simulink model "SPK_TMT_MophongSMC_4DOF"  (R2017b)
settings: Solver=FixedStepAuto  StartTime=0.0  StopTime=100  FixedStep=0.01  RelTol=1e-3
settings Model: Creator=DELL  LastModifiedBy=DELL

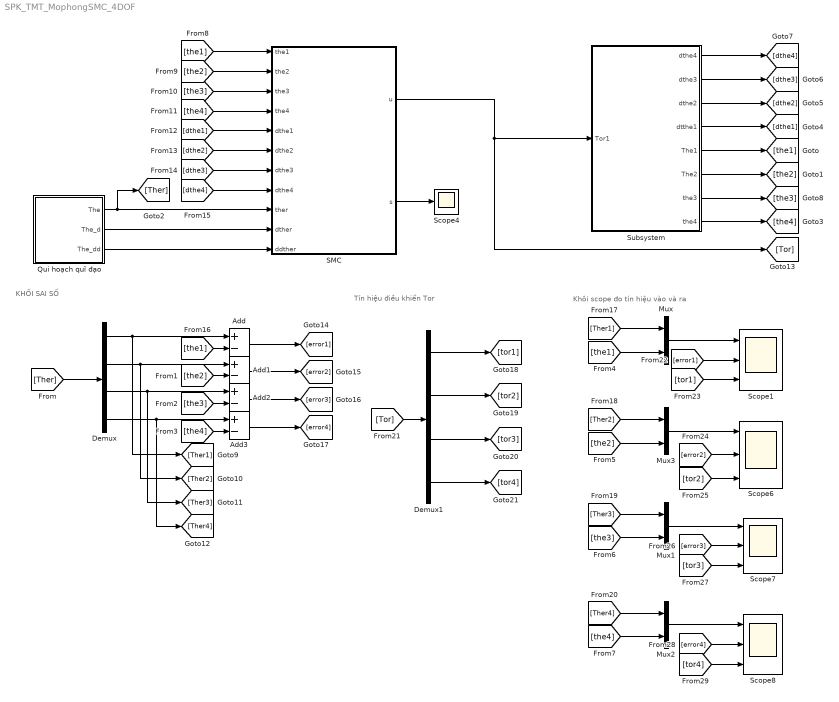
== system SPK_TMT_MophongSMC_4DOF ==
  note: Tín hiệu điều khiển Tor
  note: Khôi scope đo tín hiệu vào và ra
  note: KHỐI SAI SỐ
  Add{,1..3} (4 alike) : Sum  Inputs=+-
  Demux : Demux
  Demux1 : Demux
  Mux{,1..3} (4 alike) : Mux  Inputs=2
  "Qui hoạch quĩ đạo " : Subsystem
  SMC : MATLAB Function  TreatAsAtomicUnit=on
  Scope{1,6..8} (4 alike) : Scope  NumInputPorts=3
  Scope4 : Scope
  Subsystem : Subsystem
  wires:
  "Qui hoạch quĩ đạo "/1(The) -> [Ther], SMC/9(ther)
  "Qui hoạch quĩ đạo "/2(The_d) -> SMC/10(dther)
  "Qui hoạch quĩ đạo "/3(The_dd) -> SMC/11(ddther)
  [dthe1] -> SMC/5(dthe1)
  [the4] -> SMC/4(the4)
  [the2] -> SMC/2(the2)
  [dthe3] -> SMC/7(dthe3)
  [the1] -> SMC/1(the1)
  [dthe4] -> SMC/8(dthe4)
  [dthe2] -> SMC/6(dthe2)
  [the3] -> SMC/3(the3)
  SMC/2(s) -> Scope4/1
  Demux/1 -> [Ther1], Add/1
  [the1] -> Add/2
  Add/1 -> [error1]
  SMC/1(u) -> [Tor], Subsystem/1(Tor1)
  Subsystem/1(dthe4) -> [dthe4]
  Subsystem/2(dthe3) -> [dthe3]
  Subsystem/3(dthe2) -> [dthe2]
  Subsystem/4(dtthe1) -> [dthe1]
  Subsystem/8(the4) -> [the4]
  Subsystem/6(The2) -> [the2]
  Subsystem/5(The1) -> [the1]
  Subsystem/7(the3) -> [the3]
  [Ther] -> Demux/1
  Demux/2 -> [Ther2], Add1/1
  [the2] -> Add1/2
  Demux/3 -> [Ther3], Add2/1
  [the3] -> Add2/2
  Demux/4 -> [Ther4], Add3/1
  [the4] -> Add3/2
  Add1/1 -> [error2]
  Add2/1 -> [error3]
  Add3/1 -> [error4]
  [the1] -> Mux/2
  [the4] -> Mux2/2
  [Ther1] -> Mux/1
  [the2] -> Mux3/2
  [Ther2] -> Mux3/1
  [the3] -> Mux1/2
  [Ther3] -> Mux1/1
  [Ther4] -> Mux2/1
  Demux1/1 -> [tor1]
  Demux1/2 -> [tor2]
  Demux1/3 -> [tor3]
  Demux1/4 -> [tor4]
  [Tor] -> Demux1/1
  Mux/1 -> Scope1/1
  Mux3/1 -> Scope6/1
  Mux1/1 -> Scope7/1
  Mux2/1 -> Scope8/1
  [error1] -> Scope1/2
  [tor1] -> Scope1/3
  [error2] -> Scope6/2
  [tor2] -> Scope6/3
  [error3] -> Scope7/2
  [tor3] -> Scope7/3
  [error4] -> Scope8/2
  [tor4] -> Scope8/3

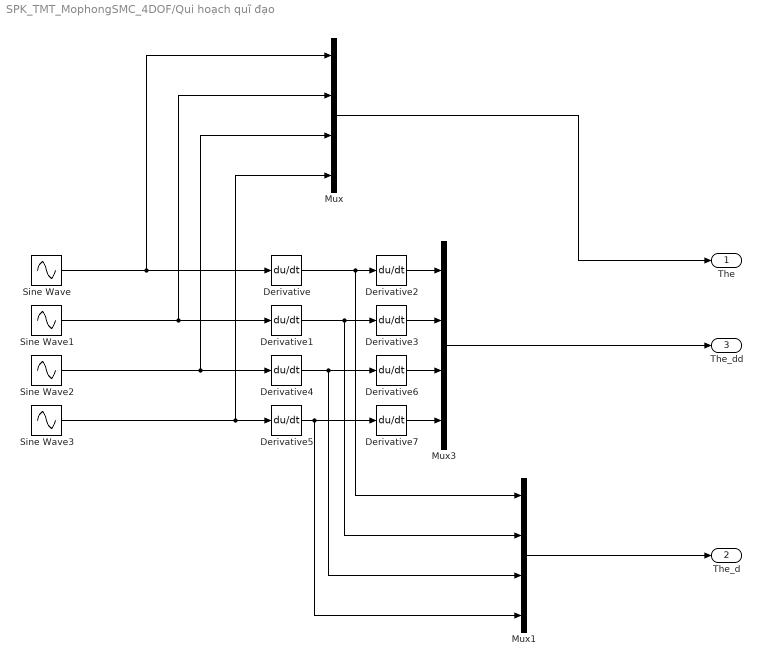
== system SPK_TMT_MophongSMC_4DOF/Qui hoạch quĩ đạo  ==
  Derivative{,1..7} (8 alike) : Derivative
  Mux : Mux
  Mux1 : Mux
  Mux3 : Mux
  Sine Wave : Sin  Amplitude=pi/6  Frequency=2*pi*0.1  SampleTime=0
  Sine Wave1 : Sin  Amplitude=pi/6  Frequency=2*pi*0.1  Phase=pi/6  SampleTime=0
  Sine Wave2 : Sin  Amplitude=pi/6  Frequency=2*pi*0.1  Phase=pi/3  SampleTime=0
  Sine Wave3 : Sin  Amplitude=pi/6  Frequency=2*pi*0.1  Phase=pi/2  SampleTime=0
  The : Outport
  The_d : Outport  Port=2
  The_dd : Outport  Port=3
  wires:
  Derivative6/1 -> Mux3/3
  Derivative7/1 -> Mux3/4
  Derivative5/1 -> Mux1/4, Derivative7/1
  Derivative4/1 -> Mux1/3, Derivative6/1
  Sine Wave2/1 -> Mux/3, Derivative4/1
  Sine Wave3/1 -> Mux/4, Derivative5/1
  Sine Wave/1 -> Mux/1, Derivative/1
  Mux1/1 -> The_d/1
  Derivative3/1 -> Mux3/2
  Derivative1/1 -> Mux1/2, Derivative3/1
  Derivative2/1 -> Mux3/1
  Sine Wave1/1 -> Mux/2, Derivative1/1
  Mux/1 -> The/1
  Mux3/1 -> The_dd/1
  Derivative/1 -> Mux1/1, Derivative2/1

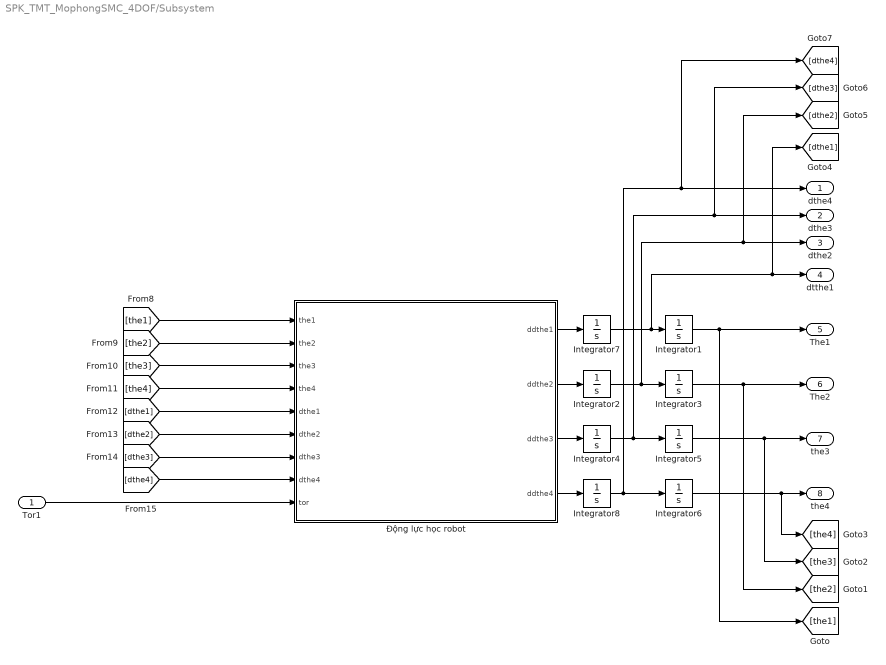
== system SPK_TMT_MophongSMC_4DOF/Subsystem ==
  Tor1 : Inport
  Integrator{1..8} (8 alike) : Integrator
  Động lực học robot : MATLAB Function  TreatAsAtomicUnit=on
  dthe4 : Outport
  dthe3 : Outport  Port=2
  dthe2 : Outport  Port=3
  dtthe1 : Outport  Port=4
  The1 : Outport  Port=5
  The2 : Outport  Port=6
  the3 : Outport  Port=7
  the4 : Outport  Port=8
  wires:
  Integrator3/1 -> [the2], The2/1
  Tor1/1 -> Động lực học robot/9(tor)
  Integrator5/1 -> [the3], the3/1
  Integrator1/1 -> [the1], The1/1
  Integrator4/1 -> [dthe3], dthe3/1, Integrator5/1
  Động lực học robot/2(ddthe2) -> Integrator2/1
  Động lực học robot/3(ddthe3) -> Integrator4/1
  Động lực học robot/4(ddthe4) -> Integrator8/1
  Integrator8/1 -> [dthe4], dthe4/1, Integrator6/1
  Động lực học robot/1(ddthe1) -> Integrator7/1
  Integrator7/1 -> [dthe1], dtthe1/1, Integrator1/1
  Integrator6/1 -> [the4], the4/1
  Integrator2/1 -> [dthe2], dthe2/1, Integrator3/1
  [dthe2] -> Động lực học robot/6(dthe2)
  [dthe4] -> Động lực học robot/8(dthe4)
  [the1] -> Động lực học robot/1(the1)
  [the2] -> Động lực học robot/2(the2)
  [the4] -> Động lực học robot/4(the4)
  [the3] -> Động lực học robot/3(the3)
  [dthe1] -> Động lực học robot/5(dthe1)
  [dthe3] -> Động lực học robot/7(dthe3)

== matlab function SPK_TMT_MophongSMC_4DOF/SMC ==
  data: the1 input; u output; the2 input; the3 input; the4 input; dthe1 input; dthe2 input; dthe3 input; dthe4 input; ther input; dther input; ddther input; s output
function [u,s]= SMC(the1, the2,the3, the4, dthe1, dthe2, dthe3, dthe4,ther,dther,ddther)
%%
m1=1;
m2=1;
m3=1;
m4=1;
L1=150;
L2=350;
L3=363.5;
L4=210;
d=140;
g=9.81;
%% M
M11=L1^2*m1 + L1^2*m2 + L1^2*m3 + (L2^2*m2)/2 + L1^2*m4 + (L2^2*m3)/2 + (L2^2*m4)/2 + (L3^2*m3)/2 + (L3^2*m4)/2 + (L4^2*m4)/2 + (L2^2*m2*cos(2*the2))/2 + (L2^2*m3*cos(2*the2))/2 + (L2^2*m4*cos(2*the2))/2 + (L4^2*m4*cos(2*the2 + 2*the3 + 2*the4))/2 + (L3^2*m3*cos(2*the2 + 2*the3))/2 + (L3^2*m4*cos(2*the2 + 2*the3))/2 + 2*L1*L3*m3*cos(the2 + the3) + 2*L1*L3*m4*cos(the2 + the3) + L2*L4*m4*cos(the3 + the4) + 2*L1*L2*m2*cos(the2) + 2*L1*L2*m3*cos(the2) + 2*L1*L2*m4*cos(the2) + L2*L3*m3*cos(the3) + L2*L3*m4*cos(the3) + L3*L4*m4*cos(the4) + L3*L4*m4*cos(2*the2 + 2*the3 + the4) + L2*L3*m3*cos(2*the2 + the3) + L2*L3*m4*cos(2*the2 + the3) + 2*L1*L4*m4*cos(the2 + the3 + the4) + L2*L4*m4*cos(2*the2 + the3 + the4);
M12=0;
M13=0;
M14=0;
M21=0;
M22=L2^2*m2 + L2^2*m3 + L2^2*m4 + L3^2*m3 + L3^2*m4 + L4^2*m4 + 2*L2*L4*m4*cos(the3 + the4) + 2*L2*L3*m3*cos(the3) + 2*L2*L3*m4*cos(the3) + 2*L3*L4*m4*cos(the4);
M23=L3^2*m3 + L3^2*m4 + L4^2*m4 + L2*L4*m4*cos(the3 + the4) + L2*L3*m3*cos(the3) + L2*L3*m4*cos(the3) + 2*L3*L4*m4*cos(the4);
M24=L4*m4*(L4 + L2*cos(the3 + the4) + L3*cos(the4));
M31=0;
M32=L3^2*m3 + L3^2*m4 + L4^2*m4 + L2*L4*m4*cos(the3 + the4) + L2*L3*m3*cos(the3) + L2*L3*m4*cos(the3) + 2*L3*L4*m4*cos(the4);
M33=L3^2*m3 + L3^2*m4 + L4^2*m4 + 2*L3*L4*m4*cos(the4);
M34=L4*m4*(L4 + L3*cos(the4));
M41=0;
M42=L4*m4*(L4 + L2*cos(the3 + the4) + L3*cos(the4));
M43=L4*m4*(L4 + L3*cos(the4));
M44=L4^2*m4;
M=[M11, M12, M13, M14;
   M21, M22, M23, M24;
   M31, M32, M33, M34;
   M41, M42, M43, M44;];

%% V
V11=- L2^2*dthe1*dthe2*m2*sin(2*the2) - L2^2*dthe1*dthe2*m3*sin(2*the2) - L2^2*dthe1*dthe2*m4*sin(2*the2) - L4^2*dthe1*dthe2*m4*sin(2*the2 + 2*the3 + 2*the4) - L4^2*dthe1*dthe3*m4*sin(2*the2 + 2*the3 + 2*the4) - L4^2*dthe1*dthe4*m4*sin(2*the2 + 2*the3 + 2*the4) - L3^2*dthe1*dthe2*m3*sin(2*the2 + 2*the3) - L3^2*dthe1*dthe2*m4*sin(2*the2 + 2*the3) - L3^2*dthe1*dthe3*m3*sin(2*the2 + 2*the3) - L3^2*dthe1*dthe3*m4*sin(2*the2 + 2*the3) - 2*L1*L2*dthe1*dthe2*m2*sin(the2) - 2*L1*L2*dthe1*dthe2*m3*sin(the2) - 2*L1*L2*dthe1*dthe2*m4*sin(the2) - L2*L3*dthe1*dthe3*m3*sin(the3) - L2*L3*dthe1*dthe3*m4*sin(the3) - L3*L4*dthe1*dthe4*m4*sin(the4) - 2*L3*L4*dthe1*dthe2*m4*sin(2*the2 + 2*the3 + the4) - 2*L3*L4*dthe1*dthe3*m4*sin(2*the2 + 2*the3 + the4) - L3*L4*dthe1*dthe4*m4*sin(2*the2 + 2*the3 + the4) - 2*L2*L3*dthe1*dthe2*m3*sin(2*the2 + the3) - 2*L2*L3*dthe1*dthe2*m4*sin(2*the2 + the3) - L2*L3*dthe1*dthe3*m3*sin(2*the2 + the3) - L2*L3*dthe1*dthe3*m4*sin(2*the2 + the3) - 2*L1*L4*dthe1*dthe2*m4*sin(the2 + the3 + the4) - 2*L1*L4*dthe1*dthe3*m4*sin(the2 + the3 + the4) - 2*L1*L4*dthe1*dthe4*m4*sin(the2 + the3 + the4) - 2*L2*L4*dthe1*dthe2*m4*sin(2*the2 + the3 + the4) - L2*L4*dthe1*dthe3*m4*sin(2*the2 + the3 + the4) - L2*L4*dthe1*dthe4*m4*sin(2*the2 + the3 + the4) - 2*L1*L3*dthe1*dthe2*m3*sin(the2 + the3) - 2*L1*L3*dthe1*dthe2*m4*sin(the2 + the3) - 2*L1*L3*dthe1*dthe3*m3*sin(the2 + the3) - 2*L1*L3*dthe1*dthe3*m4*sin(the2 + the3) - L2*L4*dthe1*dthe3*m4*sin(the3 + the4) - L2*L4*dthe1*dthe4*m4*sin(the3 + the4);
V21=(L2^2*dthe1^2*m2*sin(2*the2))/2 + (L2^2*dthe1^2*m3*sin(2*the2))/2 + (L2^2*dthe1^2*m4*sin(2*the2))/2 + (L4^2*dthe1^2*m4*sin(2*the2 + 2*the3 + 2*the4))/2 + (L3^2*dthe1^2*m3*sin(2*the2 + 2*the3))/2 + (L3^2*dthe1^2*m4*sin(2*the2 + 2*the3))/2 + L1*L2*dthe1^2*m2*sin(the2) + L1*L2*dthe1^2*m3*sin(the2) + L1*L2*dthe1^2*m4*sin(the2) - L2*L3*dthe3^2*m3*sin(the3) - L2*L3*dthe3^2*m4*sin(the3) - L3*L4*dthe4^2*m4*sin(the4) + L3*L4*dthe1^2*m4*sin(2*the2 + 2*the3 + the4) + L2*L3*dthe1^2*m3*sin(2*the2 + the3) + L2*L3*dthe1^2*m4*sin(2*the2 + the3) + L1*L4*dthe1^2*m4*sin(the2 + the3 + the4) + L2*L4*dthe1^2*m4*sin(2*the2 + the3 + the4) + L1*L3*dthe1^2*m3*sin(the2 + the3) + L1*L3*dthe1^2*m4*sin(the2 + the3) - L2*L4*dthe3^2*m4*sin(the3 + the4) - L2*L4*dthe4^2*m4*sin(the3 + the4) - 2*L2*L3*dthe2*dthe3*m3*sin(the3) - 2*L2*L3*dthe2*dthe3*m4*sin(the3) - 2*L3*L4*dthe2*dthe4*m4*sin(the4) - 2*L3*L4*dthe3*dthe4*m4*sin(the4) - 2*L2*L4*dthe2*dthe3*m4*sin(the3 + the4) - 2*L2*L4*dthe2*dthe4*m4*sin(the3 + the4) - 2*L2*L4*dthe3*dthe4*m4*sin(the3 + the4);
V31=(L4^2*dthe1^2*m4*sin(2*the2 + 2*the3 + 2*the4))/2 + (L3^2*dthe1^2*m3*sin(2*the2 + 2*the3))/2 + (L3^2*dthe1^2*m4*sin(2*the2 + 2*the3))/2 + (L2*L3*dthe1^2*m3*sin(the3))/2 + (L2*L3*dthe1^2*m4*sin(the3))/2 + L2*L3*dthe2^2*m3*sin(the3) + L2*L3*dthe2^2*m4*sin(the3) - L3*L4*dthe4^2*m4*sin(the4) + L3*L4*dthe1^2*m4*sin(2*the2 + 2*the3 + the4) + (L2*L3*dthe1^2*m3*sin(2*the2 + the3))/2 + (L2*L3*dthe1^2*m4*sin(2*the2 + the3))/2 + L1*L4*dthe1^2*m4*sin(the2 + the3 + the4) + (L2*L4*dthe1^2*m4*sin(2*the2 + the3 + the4))/2 + L1*L3*dthe1^2*m3*sin(the2 + the3) + L1*L3*dthe1^2*m4*sin(the2 + the3) + (L2*L4*dthe1^2*m4*sin(the3 + the4))/2 + L2*L4*dthe2^2*m4*sin(the3 + the4) - 2*L3*L4*dthe2*dthe4*m4*sin(the4) - 2*L3*L4*dthe3*dthe4*m4*sin(the4);
V41=(L4*m4*(L2*dthe1^2*sin(the3 + the4) + 2*L2*dthe2^2*sin(the3 + the4) + L3*dthe1^2*sin(the4) + 2*L3*dthe2^2*sin(the4) + 2*L3*dthe3^2*sin(the4) + L3*dthe1^2*sin(2*the2 + 2*the3 + the4) + 2*L1*dthe1^2*sin(the2 + the3 + the4) + L4*dthe1^2*sin(2*the2 + 2*the3 + 2*the4) + L2*dthe1^2*sin(2*the2 + the3 + the4) + 4*L3*dthe2*dthe3*sin(the4)))/2;
V=[V11;V21;V31;V41];
%% G
G11=0;
G21=- g*m4*(L3*cos(the2 + the3) + L2*cos(the2) + L4*cos(the2 + the3 + the4)) - g*m3*(L3*cos(the2 + the3) + L2*cos(the2)) - L2*g*m2*cos(the2);
G31=- g*m4*(L3*cos(the2 + the3) + L4*cos(the2 + the3 + the4)) - L3*g*m3*cos(the2 + the3);
G41=-L4*g*m4*cos(the2 + the3 + the4);
G=[G11; G21; G31; G41];
%% Control
the=[the1;the2;the3;the4];
the_dot=[dthe1; dthe2; dthe3; dthe4];
lamla=150;
K=40;
eta=10;
% lamla=30;
% K=40;
% eta=10;
fx=-inv(M)*(V+G);
gx=inv(M);

E=the-ther;
dE=the_dot-dther;
s=lamla*E+dE;
u=inv(gx)*(ddther-lamla*dE-fx-K*s-eta*sign(s))
end

== matlab function SPK_TMT_MophongSMC_4DOF/Subsystem/Động lực học robot ==
  data: the1 input; ddthe1 output; the2 input; the3 input; the4 input; dthe1 input; dthe2 input; dthe3 input; dthe4 input; tor input; ddthe2 output; ddthe3 output; ddthe4 output
function [ddthe1, ddthe2, ddthe3, ddthe4]= fcn(the1, the2,the3, the4, dthe1, dthe2, dthe3, dthe4,tor)
%% Thông số
m1=1;
m2=1;
m3=1;
m4=1;
L1=150;
L2=350;
L3=363.5;
L4=210;
d=140;
g=9.81;

%% M
M11=L1^2*m1 + L1^2*m2 + L1^2*m3 + (L2^2*m2)/2 + L1^2*m4 + (L2^2*m3)/2 + (L2^2*m4)/2 + (L3^2*m3)/2 + (L3^2*m4)/2 + (L4^2*m4)/2 + (L2^2*m2*cos(2*the2))/2 + (L2^2*m3*cos(2*the2))/2 + (L2^2*m4*cos(2*the2))/2 + (L4^2*m4*cos(2*the2 + 2*the3 + 2*the4))/2 + (L3^2*m3*cos(2*the2 + 2*the3))/2 + (L3^2*m4*cos(2*the2 + 2*the3))/2 + 2*L1*L3*m3*cos(the2 + the3) + 2*L1*L3*m4*cos(the2 + the3) + L2*L4*m4*cos(the3 + the4) + 2*L1*L2*m2*cos(the2) + 2*L1*L2*m3*cos(the2) + 2*L1*L2*m4*cos(the2) + L2*L3*m3*cos(the3) + L2*L3*m4*cos(the3) + L3*L4*m4*cos(the4) + L3*L4*m4*cos(2*the2 + 2*the3 + the4) + L2*L3*m3*cos(2*the2 + the3) + L2*L3*m4*cos(2*the2 + the3) + 2*L1*L4*m4*cos(the2 + the3 + the4) + L2*L4*m4*cos(2*the2 + the3 + the4);
M12=0;
M13=0;
M14=0;
M21=0;
M22=L2^2*m2 + L2^2*m3 + L2^2*m4 + L3^2*m3 + L3^2*m4 + L4^2*m4 + 2*L2*L4*m4*cos(the3 + the4) + 2*L2*L3*m3*cos(the3) + 2*L2*L3*m4*cos(the3) + 2*L3*L4*m4*cos(the4);
M23=L3^2*m3 + L3^2*m4 + L4^2*m4 + L2*L4*m4*cos(the3 + the4) + L2*L3*m3*cos(the3) + L2*L3*m4*cos(the3) + 2*L3*L4*m4*cos(the4);
M24=L4*m4*(L4 + L2*cos(the3 + the4) + L3*cos(the4));
M31=0;
M32=L3^2*m3 + L3^2*m4 + L4^2*m4 + L2*L4*m4*cos(the3 + the4) + L2*L3*m3*cos(the3) + L2*L3*m4*cos(the3) + 2*L3*L4*m4*cos(the4);
M33=L3^2*m3 + L3^2*m4 + L4^2*m4 + 2*L3*L4*m4*cos(the4);
M34=L4*m4*(L4 + L3*cos(the4));
M41=0;
M42=L4*m4*(L4 + L2*cos(the3 + the4) + L3*cos(the4));
M43=L4*m4*(L4 + L3*cos(the4));
M44=L4^2*m4;
M=[M11, M12, M13, M14;
   M21, M22, M23, M24;
   M31, M32, M33, M34;
   M41, M42, M43, M44;];

%% V
V11=- L2^2*dthe1*dthe2*m2*sin(2*the2) - L2^2*dthe1*dthe2*m3*sin(2*the2) - L2^2*dthe1*dthe2*m4*sin(2*the2) - L4^2*dthe1*dthe2*m4*sin(2*the2 + 2*the3 + 2*the4) - L4^2*dthe1*dthe3*m4*sin(2*the2 + 2*the3 + 2*the4) - L4^2*dthe1*dthe4*m4*sin(2*the2 + 2*the3 + 2*the4) - L3^2*dthe1*dthe2*m3*sin(2*the2 + 2*the3) - L3^2*dthe1*dthe2*m4*sin(2*the2 + 2*the3) - L3^2*dthe1*dthe3*m3*sin(2*the2 + 2*the3) - L3^2*dthe1*dthe3*m4*sin(2*the2 + 2*the3) - 2*L1*L2*dthe1*dthe2*m2*sin(the2) - 2*L1*L2*dthe1*dthe2*m3*sin(the2) - 2*L1*L2*dthe1*dthe2*m4*sin(the2) - L2*L3*dthe1*dthe3*m3*sin(the3) - L2*L3*dthe1*dthe3*m4*sin(the3) - L3*L4*dthe1*dthe4*m4*sin(the4) - 2*L3*L4*dthe1*dthe2*m4*sin(2*the2 + 2*the3 + the4) - 2*L3*L4*dthe1*dthe3*m4*sin(2*the2 + 2*the3 + the4) - L3*L4*dthe1*dthe4*m4*sin(2*the2 + 2*the3 + the4) - 2*L2*L3*dthe1*dthe2*m3*sin(2*the2 + the3) - 2*L2*L3*dthe1*dthe2*m4*sin(2*the2 + the3) - L2*L3*dthe1*dthe3*m3*sin(2*the2 + the3) - L2*L3*dthe1*dthe3*m4*sin(2*the2 + the3) - 2*L1*L4*dthe1*dthe2*m4*sin(the2 + the3 + the4) - 2*L1*L4*dthe1*dthe3*m4*sin(the2 + the3 + the4) - 2*L1*L4*dthe1*dthe4*m4*sin(the2 + the3 + the4) - 2*L2*L4*dthe1*dthe2*m4*sin(2*the2 + the3 + the4) - L2*L4*dthe1*dthe3*m4*sin(2*the2 + the3 + the4) - L2*L4*dthe1*dthe4*m4*sin(2*the2 + the3 + the4) - 2*L1*L3*dthe1*dthe2*m3*sin(the2 + the3) - 2*L1*L3*dthe1*dthe2*m4*sin(the2 + the3) - 2*L1*L3*dthe1*dthe3*m3*sin(the2 + the3) - 2*L1*L3*dthe1*dthe3*m4*sin(the2 + the3) - L2*L4*dthe1*dthe3*m4*sin(the3 + the4) - L2*L4*dthe1*dthe4*m4*sin(the3 + the4);
V21=(L2^2*dthe1^2*m2*sin(2*the2))/2 + (L2^2*dthe1^2*m3*sin(2*the2))/2 + (L2^2*dthe1^2*m4*sin(2*the2))/2 + (L4^2*dthe1^2*m4*sin(2*the2 + 2*the3 + 2*the4))/2 + (L3^2*dthe1^2*m3*sin(2*the2 + 2*the3))/2 + (L3^2*dthe1^2*m4*sin(2*the2 + 2*the3))/2 + L1*L2*dthe1^2*m2*sin(the2) + L1*L2*dthe1^2*m3*sin(the2) + L1*L2*dthe1^2*m4*sin(the2) - L2*L3*dthe3^2*m3*sin(the3) - L2*L3*dthe3^2*m4*sin(the3) - L3*L4*dthe4^2*m4*sin(the4) + L3*L4*dthe1^2*m4*sin(2*the2 + 2*the3 + the4) + L2*L3*dthe1^2*m3*sin(2*the2 + the3) + L2*L3*dthe1^2*m4*sin(2*the2 + the3) + L1*L4*dthe1^2*m4*sin(the2 + the3 + the4) + L2*L4*dthe1^2*m4*sin(2*the2 + the3 + the4) + L1*L3*dthe1^2*m3*sin(the2 + the3) + L1*L3*dthe1^2*m4*sin(the2 + the3) - L2*L4*dthe3^2*m4*sin(the3 + the4) - L2*L4*dthe4^2*m4*sin(the3 + the4) - 2*L2*L3*dthe2*dthe3*m3*sin(the3) - 2*L2*L3*dthe2*dthe3*m4*sin(the3) - 2*L3*L4*dthe2*dthe4*m4*sin(the4) - 2*L3*L4*dthe3*dthe4*m4*sin(the4) - 2*L2*L4*dthe2*dthe3*m4*sin(the3 + the4) - 2*L2*L4*dthe2*dthe4*m4*sin(the3 + the4) - 2*L2*L4*dthe3*dthe4*m4*sin(the3 + the4);
V31=(L4^2*dthe1^2*m4*sin(2*the2 + 2*the3 + 2*the4))/2 + (L3^2*dthe1^2*m3*sin(2*the2 + 2*the3))/2 + (L3^2*dthe1^2*m4*sin(2*the2 + 2*the3))/2 + (L2*L3*dthe1^2*m3*sin(the3))/2 + (L2*L3*dthe1^2*m4*sin(the3))/2 + L2*L3*dthe2^2*m3*sin(the3) + L2*L3*dthe2^2*m4*sin(the3) - L3*L4*dthe4^2*m4*sin(the4) + L3*L4*dthe1^2*m4*sin(2*the2 + 2*the3 + the4) + (L2*L3*dthe1^2*m3*sin(2*the2 + the3))/2 + (L2*L3*dthe1^2*m4*sin(2*the2 + the3))/2 + L1*L4*dthe1^2*m4*sin(the2 + the3 + the4) + (L2*L4*dthe1^2*m4*sin(2*the2 + the3 + the4))/2 + L1*L3*dthe1^2*m3*sin(the2 + the3) + L1*L3*dthe1^2*m4*sin(the2 + the3) + (L2*L4*dthe1^2*m4*sin(the3 + the4))/2 + L2*L4*dthe2^2*m4*sin(the3 + the4) - 2*L3*L4*dthe2*dthe4*m4*sin(the4) - 2*L3*L4*dthe3*dthe4*m4*sin(the4);
V41=(L4*m4*(L2*dthe1^2*sin(the3 + the4) + 2*L2*dthe2^2*sin(the3 + the4) + L3*dthe1^2*sin(the4) + 2*L3*dthe2^2*sin(the4) + 2*L3*dthe3^2*sin(the4) + L3*dthe1^2*sin(2*the2 + 2*the3 + the4) + 2*L1*dthe1^2*sin(the2 + the3 + the4) + L4*dthe1^2*sin(2*the2 + 2*the3 + 2*the4) + L2*dthe1^2*sin(2*the2 + the3 + the4) + 4*L3*dthe2*dthe3*sin(the4)))/2;
V=[V11;V21;V31;V41];
%% G
G11=0;
G21=- g*m4*(L3*cos(the2 + the3) + L2*cos(the2) + L4*cos(the2 + the3 + the4)) - g*m3*(L3*cos(the2 + the3) + L2*cos(the2)) - L2*g*m2*cos(the2);
G31=- g*m4*(L3*cos(the2 + the3) + L4*cos(the2 + the3 + the4)) - L3*g*m3*cos(the2 + the3);
G41=-L4*g*m4*cos(the2 + the3 + the4);
G=[G11; G21; G31; G41];
%% Tính theta2dd
ddtheta=inv(M)*(tor-V-G);
%-diag([4;4;4;4])*[dthe1; dthe2; dthe3; dthe4]);
ddthe1=ddtheta(1);
ddthe2=ddtheta(2);
ddthe3=ddtheta(3);
ddthe4=ddtheta(4);
end
